simulink model "gvn"  (R2022b)
settings: Solver=VariableStepAuto  StartTime=0.0  StopTime=10.0  RelTol=1e-3
InitFcn:
  | % PARÁMETROS
  | L=12e-3;R=20;r=0.3;d=3.5;kt=0.5;kb=0.01;J=0.002;b=1.2;b2=1.7;
  | Mp=110;Me=110; M = Mp + Me; g = 0;
  | d=3.5; ref = 1*d; %SUBIR UN PISO
  | % MATRICES DEL SISTEMA
  | A=[-R/L,0,-kb/L/r;0,0,1;kt*r/(M*r^2+J),0,-(r^2*b2+b)/(M*r^2+J)];
  | B=[1/L;0;0];
  | C = [0 1 0];
  | V = [0;0;-r^2*M*g/(M*r^2+J)];
  | % Diseño del controlador
  | Mc=[B,A*B,A^2*B];
  | Ha=(A-pd(1)*eye(3))*(A-pd(2)*eye(3))*(A-pd(3)*eye(3));
  | K=real(-[0 0 1]*Mc^-1*Ha);
  | F=real((C*(-A-B*K)^-1*B)^-1); %CASO 1
  | %F=real((C*(-A-B*K)^-1*B*ref)^-1*(ref-C*(-A-B*K)^-1*V)); %CASO 2
  | %F=real((C*(-Ac-B*K)^-1*B*ref)^-1*(ref-C*(-Ac-B*K)^-1*Vc)); %CASO 3; %CASO 3
settings Model: Creator=garci  LastModifiedBy=garci

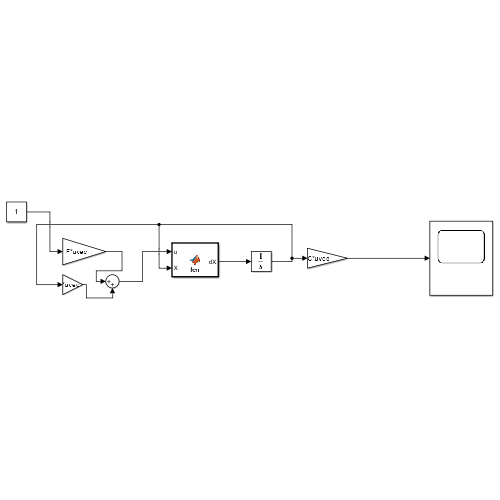
[thumbnail: Simulink's stored preview of the top-level diagram]
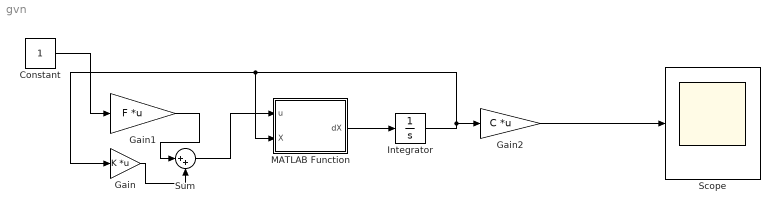
== system gvn ==
  Constant : Constant
  Gain : Gain  Gain=K  Multiplication=Matrix(K*u) (u vector)
  Gain1 : Gain  Gain=F  Multiplication=Matrix(K*u) (u vector)
  Gain2 : Gain  Gain=C  Multiplication=Matrix(K*u) (u vector)
  Integrator : Integrator  InitialCondition=[0;0;0]
  MATLAB Function : MATLAB Function  TreatAsAtomicUnit=on
  Scope : Scope
  Sum : Sum  Inputs=|++
  wires:
  Gain/1 -> Sum/2
  Gain1/1 -> Sum/1
  Constant/1 -> Gain1/1
  MATLAB Function/1(dX) -> Integrator/1
  Integrator/1 -> Gain/1, MATLAB Function/2(X), Gain2/1
  Sum/1 -> MATLAB Function/1(u)
  Gain2/1 -> Scope/1

== matlab function gvn/MATLAB Function ==
  data: u input; X input; dX output; A parameter; B parameter; V parameter
function dX = fcn(u,X,A,B,V)
dX = A*X+B*u+V;
